simulink model "ejercicio2"  (R2024b)
settings: Solver=VariableStepAuto  StartTime=0.0  StopTime=5  RelTol=1e-3
settings Model: Creator=david  LastModifiedBy=david
settings DataIOCC: ReturnWorkspaceOutputs=off

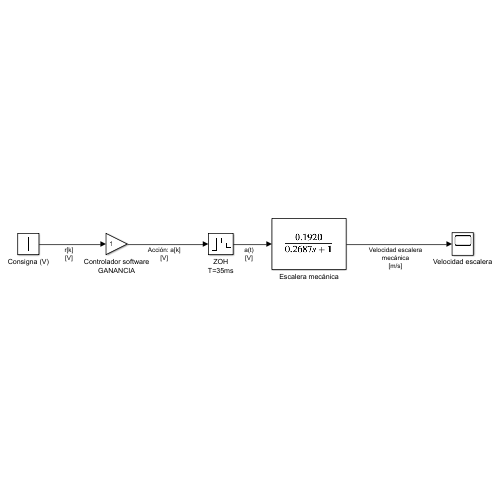
[thumbnail: Simulink's stored preview of the top-level diagram]
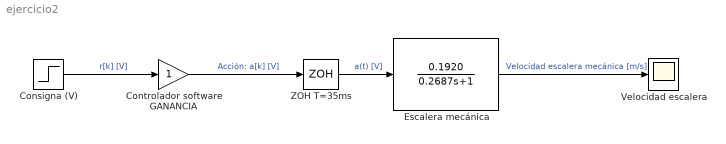
== system ejercicio2 ==
  Consigna (V) : Step  Time=0  SampleTime=0
  Controlador software GANANCIA : Gain
  Escalera mecánica : TransferFcn  Numerator=0.1920  Denominator=[0.2687 1]
  Velocidad escalera : Scope
  ZOH T=35ms : ZeroOrderHold  SampleTime=35e-3
  wires:
  Consigna (V)/1 -> Controlador software GANANCIA/1  "r[k] [V]"
  Controlador software GANANCIA/1 -> ZOH T=35ms/1  "Acción: a[k] [V]"
  ZOH T=35ms/1 -> Escalera mecánica/1  "a(t) [V]"
  Escalera mecánica/1 -> Velocidad escalera/1  "Velocidad escalera mecánica [m/s]"
